simulink model "model"  (R2020a)
settings: Solver=VariableStepAuto  StartTime=0.0  StopTime=inf  RelTol=1e-3
undefined symbols (not defined in the file): f
libraries: instrumentlib x2, aerolibanimutils x1
settings Model: Creator=User  LastModifiedBy=yasiu

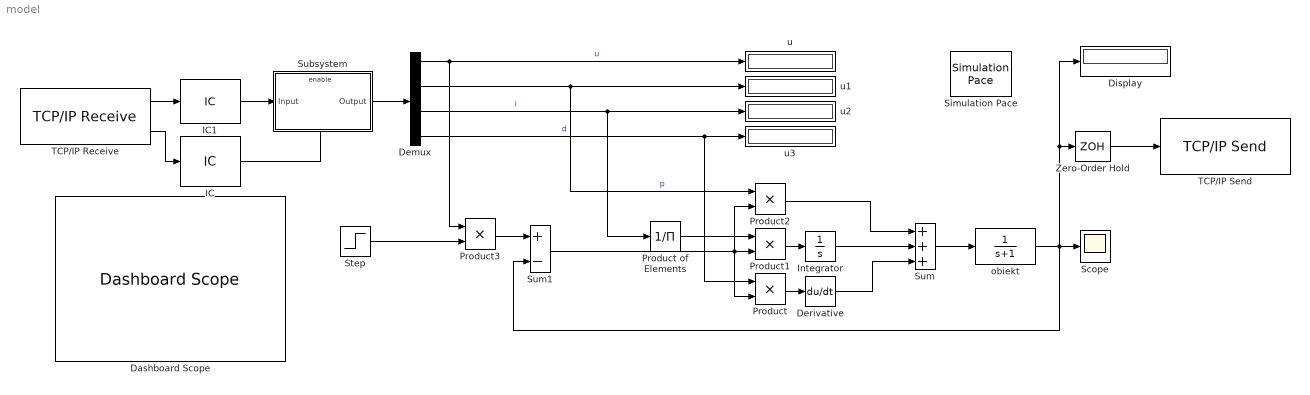
== system model ==
  Dashboard Scope : DashboardScope  Ymin=-5  Ymax=5  ScaleAtStop=off
  Demux : Demux
  Derivative : Derivative
  Display : Display
  IC : InitialCondition
  IC1 : InitialCondition  Value=[1;1;1;1]
  Integrator : Integrator
  Product{,1..3} (4 alike) : Product
  Product of Elements : Product  Inputs=/
  Scope : Scope
  Simulation Pace : aerolibanimutils/Simulation Pace  SimulationPace=1  SleepMode=Auto  OutputPaceError=off  SampleTime=0.1
  Step : Step  SampleTime=0
  Subsystem : Subsystem
  Sum : Sum  Inputs=+++
  Sum1 : Sum  Inputs=+-
  TCP/IP Receive : instrumentlib/TCP//IP Receive  Host=192.168.1.104  Port=5555  DataSize=4  EnableBlockingMode=off  Timeout=10  SampleTime=0.01  DataType=double  ByteOrder=BigEndian  ASCIIFormatting=%f,  Terminator=LF
  TCP/IP Send : instrumentlib/TCP//IP Send  Host=192.168.1.104  Port=5555  EnableBlockingMode=off  Timeout=10  ByteOrder=BigEndian  TransferDelay=off
  Zero-Order Hold : ZeroOrderHold  SampleTime=0.1
  obiekt : TransferFcn  Denominator=[1 1]
  u{,1..3} (4 alike) : Display
  wires:
  Product/1 -> Derivative/1
  Product1/1 -> Integrator/1
  Product2/1 -> Sum/1
  Integrator/1 -> Sum/2
  Derivative/1 -> Sum/3
  Sum1/1 -> Product2/2, Product/2, Product1/2
  Sum/1 -> obiekt/1
  obiekt/1 -> Display/1, Zero-Order Hold/1, Scope/1, Sum1/2
  Product3/1 -> Sum1/1
  Demux/1 -> Product3/1, u/1  "u"
  Demux/2 -> Product2/1, u1/1  "p"
  Demux/3 -> Product of Elements/1, u2/1  "i"
  Demux/4 -> Product/1, u3/1  "d"
  TCP/IP Receive/1 -> IC1/1
  TCP/IP Receive/2 -> IC/1
  Subsystem/1(Output) -> Demux/1
  IC/1 -> Subsystem/Enable
  IC1/1 -> Subsystem/1(Input)
  Product of Elements/1 -> Product1/1
  Zero-Order Hold/1 -> TCP/IP Send/1
  Step/1 -> Product3/2

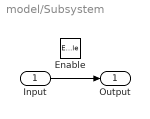
== system model/Subsystem ==
  Input : Inport
  Enable : EnablePort
  Output : Outport
  wires:
  Input/1 -> Output/1
